simulink model "flexcan_s32k11x"  (Simulink 9.0)
settings: Solver=FixedStepDiscrete  StartTime=0.0  StopTime=10.0  FixedStep=0.1  RelTol=1e-3  EnableMultiTasking=on
InitFcn:
  | mbd_s32k_consistency_checks(bdroot(gcs));
undefined symbols (not defined in the file): LQFP, thumb
libraries: mbd_s32k1xx_ec_toolbox x9, simulink x1
Description:
  | This model tests the FlexCAN communication.
  | A numeric sequence with ID 0x3FF is send continuosly on FlexCAN0 to test the busload.
  | A received message with ID 0x3FE will toggle the PTD15 pin (Red LED) on each receive.
  | 
  | HW prerequisite:
  | - S32K116EVB-Q048/S32K118EVB
  | - Make sure that J107 has pin 1 and 2 connected and external power supply is provieded through J16.
  | 
  | Validation:
  | - The CAN Baudrate is set to 500 Kb/s.
  | - Any CAN analizer (USB to CAN device) can be used to observe CAN traffic via board CAN port J13.
settings Model: Creator=NXP MBDT Team  LastModifiedBy=nxf35401
settings DataIOCC: ExternalInput=off  InitialState=off  LimitDataPoints=on  SaveOutput=off  SignalLogging=off  SaveTime=off
settings OptimizationCC: DefaultParameterBehavior=Inlined  EnhancedBackFolding=on  PassReuseOutputArgsAs=Individual arguments  LifeSpan=auto  OptimizeBlockOrder=speed  DifferentSizesBufferReuse=on
settings DebuggingCC: SolverPrmCheckMsg=warning  InheritedTsInSrcMsg=none  SingleTaskRateTransMsg=error  ParameterTunabilityLossMsg=error  UnconnectedInputMsg=error  UnconnectedOutputMsg=error  UnconnectedLineMsg=error  AllowSymbolicDim=off  UnknownTsInhSupMsg=error  StateNameClashWarn=warning
settings HardwareCC: ProdLargestAtomicInteger=Long  ProdLargestAtomicFloat=Double  ProdIntDivRoundTo=Zero  ProdEndianess=LittleEndian  ProdHWDeviceType=ARM Compatible->ARM Cortex
settings SFSimCC: MATLABDynamicMemAlloc=off
settings RTWCC: SystemTargetFile=mbd_s32k.tlc  MakeCommand=mbd_s32k_make_rtw COPY_MDLREF_INCLUDES=0  TemplateMakefile=mbd_s32k.tmf  Description=Model Based Design Toolbox S32K14x Code Generation Target  GenerateReport=on  IncludeHyperlinkInReport=on  LaunchReport=on  GenerateTraceInfo=on  GenerateTraceReport=on  GenerateTraceReportSl=on  GenerateTraceReportSf=on  GenerateTraceReportEml=on
settings CodeAppCC: ForceParamTrailComments=on  IgnoreCustomStorageClasses=off  OperatorAnnotations=on  SimulinkDataObjDesc=on  SFDataObjDesc=on  InsertBlockDesc=on  StateflowObjectComments=off
settings STFCustomTargetCC: MultiwordLength=256  ModelReferenceCompliant=off  CombineOutputUpdateFcns=on  ERTCustomFileBanners=on  SupportContinuousTime=off  SupportNonInlinedSFcns=off  RemoveResetFunc=on  MATLABClassNameForMDSCustomization=Simulink.SoftwareTarget.ERTCustomization  GRTInterface=off  SystemTargetFile=mbd_s32k.tlc
settings ERTTargetCC: ModelReferenceCompliant=off  ParMdlRefBuildCompliant=off  CompOptLevelCompliant=off  ConcurrentExecutionCompliant=off  ModelStepFunctionPrototypeControlCompliant=off  CPPClassGenCompliant=off  UseToolchainInfoCompliant=off  InlinedParameterPlacement=NonHierarchical  ERTCustomFileTemplate=example_file_process.tlc

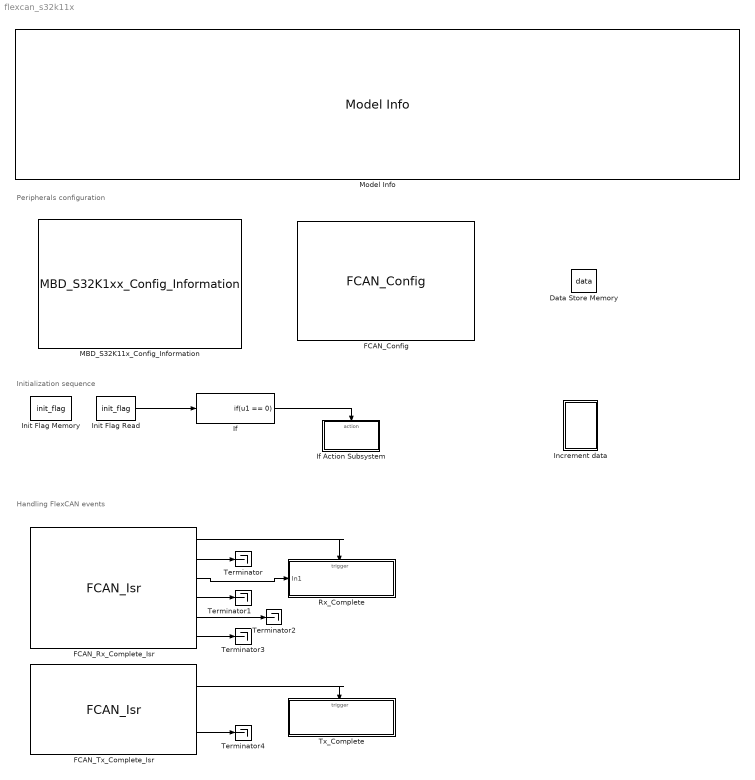
== system flexcan_s32k11x ==
  note: Peripherals configuration
  note: Handling FlexCAN events
  note: Initialization sequence
  Data Store Memory : DataStoreMemory  DataStoreName=data  ReadBeforeWriteMsg=warning  WriteAfterWriteMsg=warning  WriteAfterReadMsg=warning  ShowAdditionalParam=off  OutDataTypeStr=uint8
  FCAN_Config : mbd_s32k1xx_ec_toolbox/Communication Blocks/CAN Blocks/FCAN_Config  Priority=1  can_instance=0  can_mode=Normal mode  can_max_num_mb=16  can_rx=PTE4: [CAN0_RX | CAN Rx channel]  can_tx=PTE5: [CAN0_TX | CAN Tx Channel]  show_adv_opts=on  can_clk_src=Peripheral clock  bitrate=500  bitrate_adv_opts=off  can_presdiv=3  can_rjw=3  can_pseg1=6  can_pseg2=3  can_propseg=7  can_cbt_presdiv=1  can_cbt_rjw=3  can_cbt_pseg1=7  can_cbt_pseg2=7  can_cbt_propseg=6  can_fd_enable=off  can_payload=8  can_rxfifo_enable=off  can_fifo_id_filter_extended=off  can_fifo_id_filter_remote=off  can_num_id_filters=8  can_fifo_id_format=A  can_fifo_id_filter={'0x0', '0x0', '0x0', '0x0', '0x0', '0x0', '0x0', '0x0'}  can_pn_enable=off  can_wakeup_match=off  can_wakeup_timeout=off  can_timeout_en=off  can_match_timeout=1  can_multiple_matches_en=off  can_num_matches=1  can_idfilter_extendedid=off  can_idfilter_remoteframe=off  can_idfilter_type=Match exact  can_idfilter_id1=0  can_idfilter_id2=0  can_payloadfilter_enable=off  can_payloadfilter_dlclow=0  can_payloadfilter_dlchigh=0  can_payloadfilter_type=Match exact  can_payloadfilter_payload1_b0=0  can_payloadfilter_payload1_b1=0  can_payloadfilter_payload1_b2=0  can_payloadfilter_payload1_b3=0  can_payloadfilter_payload1_b4=0  can_payloadfilter_payload1_b5=0  can_payloadfilter_payload1_b6=0  can_payloadfilter_payload1_b7=0  can_payloadfilter_payload2_b0=0  can_payloadfilter_payload2_b1=0  can_payloadfilter_payload2_b2=0  can_payloadfilter_payload2_b3=0  can_payloadfilter_payload2_b4=0  can_payloadfilter_payload2_b5=0  can_payloadfilter_payload2_b6=0  can_payloadfilter_payload2_b7=0
  FCAN_Rx_Complete_Isr : mbd_s32k1xx_ec_toolbox/Communication Blocks/CAN Blocks/FCAN_Isr  can_instance=0  can_event=Rx Complete
  FCAN_Tx_Complete_Isr : mbd_s32k1xx_ec_toolbox/Communication Blocks/CAN Blocks/FCAN_Isr  can_instance=0  can_event=Tx Complete
  If : If  IfExpression=u1 == 0  ShowElse=off
  If Action Subsystem : Subsystem  TreatAsAtomicUnit=on
  Increment data : Subsystem
  Init Flag Memory : DataStoreMemory  DataStoreName=init_flag  ReadBeforeWriteMsg=warning  WriteAfterWriteMsg=warning  WriteAfterReadMsg=warning  ShowAdditionalParam=off  OutDataTypeStr=uint32
  Init Flag Read : DataStoreRead  DataStoreName=init_flag
  MBD_S32K11x_Config_Information : mbd_s32k1xx_ec_toolbox/MBD_S32K1xx_Config_Information  mbdt_ver=0  disp_str=|  config_params=[]  mcu_target_name=S32K116  mcu_target_package=48-LQFP  mcu_target_sram_size=17KB  mcu_system_clock_freq=40  mcu_xtal_freq=External 40  mcu_steptick_timer=LPIT Channel 0  mcu_steptick_prio=3  ds_import_enable=on  target_compiler=GCC  target_memory=FLASH  gcc_target_compile_opts=-mcpu=cortex-m0plus -mthumb -O1 -g -gstrict-dwarf  gcc_target_assemble_opts=-mcpu=cortex-m0plus -mthumb -g  gcc_target_link_opts=-mcpu=cortex-m0plus -mthumb  gcc_target_default_lcf=on  gcc_target_user_lcf=S32K116_17_flash.ld  ghs_target_compile_opts=-thumb -Ogeneral -Wundef -Wimplicit-int -Wshadow -Wtrigraphs --no_commons -c99 --gnu_asm -gdwarf-2 -G  ghs_target_assemble_opts=-thumb -preprocess_assembly_files -fsoft --gnu_asm  ghs_target_link_opts=-thumb  ghs_target_default_lcf=on  ghs_target_user_lcf=S32K116_17_flash.ld  iar_target_compile_opts=--thumb -Ol -e --debug --dlib_config normal  iar_target_assemble_opts=--thumb  iar_target_link_opts=--no_exceptions --vfe --inline  iar_target_default_lcf=on  iar_target_user_lcf=S32K116_17_flash.icf  pil_download_enable=off  rbl_download_enable=on  rbl_start_delay=5000  rbl_download_interface=OpenSDA  rbl_restart_request=off  rbl_com_port=Custom  rbl_com_port_custom=COM1  pil_download_rate=57600  pil_opensda_drive=Custom  pil_opensda_drive_custom=D  pil_uart_instance=0  pil_uart_rx=PTB0: [LPUART0_RX | Receive]  pil_uart_tx=PTB1: [LPUART0_TX | Transmit]  FTM_PWM_PcrCheckEnDis=on  FTM_Input_Edge_Inputs_PcrCheckEnDis=on  FTM_Dual_Edge_Inputs_PcrCheckEnDis=on  FTM_Quadrature_Inputs_PcrCheckEnDis=on  FTM_Hall_Sensor_Inputs_PcrCheckEnDis=on  LPTMR_PcrCheckEnDis=on  PIT_PcrCheckEnDis=on  RTC_PcrCheckEnDis=on  FlexCAN_PcrCheckEnDis=on  LIN_PcrCheckEnDis=on  FlexIO_PcrCheckEnDis=on  LPI2C_PcrCheckEnDis=on  LPSPI_PcrCheckEnDis=on  LPUART_PcrCheckEnDis=on  CMP_PcrCheckEnDis=on  GPIO_OutputPcrCheckEnDis=on  GPIO_InputPcrCheckEnDis=on  SBC_PcrCheckEnDis=on  AMMCLIB_PcrCheckEnDis=on  FM_PcrCheckEnDis=on  Profile_PcrCheckEnDis=on  ConfigParams_PcrCheckEnDis=on  ModelRef_PcrCheckEnDis=on  PDB0_PcrCheckEnDis=on  CSEc_PcrCheckEnDis=on  eDMA_PcrCheckEnDis=on  ADC_PcrCheckEnDis=on  WDOG_PcrCheckEnDis=on
      | Target : S32K144-64KB_SRAM
      | Package : 100-pin
      | System clock : 80 MHz
      | XTAL clock : External 8 MHz
      | Compiler : IAR
      | Target Type : FLASH
      | Download Code after build : off
      | Step Tick Interrupt Priority : 15
  Model Info : simulink/Model-Wide Utilities/Model Info  Frame=on  DisplayStringWithTags=|  HorizontalTextAlignment=Left  LeftAlignmentValue=0.02
      | Model Name: %<ModelName>
      | 
      | Description: %<Description>
  Rx_Complete : Subsystem  TreatAsAtomicUnit=on
      settings: RTWSystemCode=Nonreusable function
  Terminator{,1..4} (5 alike) : Terminator
  Tx_Complete : Subsystem  TreatAsAtomicUnit=on
      settings: RTWSystemCode=Nonreusable function
  wires:
  If/1 -> If Action Subsystem/Action
  Init Flag Read/1 -> If/1
  FCAN_Rx_Complete_Isr/1 -> Rx_Complete/Trigger
  FCAN_Rx_Complete_Isr/3 -> Rx_Complete/1(In1)
  FCAN_Tx_Complete_Isr/1 -> Tx_Complete/Trigger
  FCAN_Rx_Complete_Isr/2 -> Terminator/1
  FCAN_Rx_Complete_Isr/4 -> Terminator1/1
  FCAN_Rx_Complete_Isr/5 -> Terminator2/1
  FCAN_Tx_Complete_Isr/2 -> Terminator4/1
  FCAN_Rx_Complete_Isr/6 -> Terminator3/1

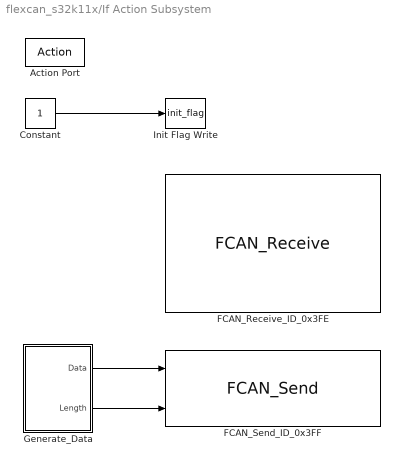
== system flexcan_s32k11x/If Action Subsystem ==
  Action Port : ActionPort  ActionType=then
  Constant : Constant  OutDataTypeStr=uint32
  FCAN_Receive_ID_0x3FE : mbd_s32k1xx_ec_toolbox/Communication Blocks/CAN Blocks/FCAN_Receive  can_instance=0  can_mode=Non-blocking  can_timeout_ms=0  can_mb_idx=14  can_extended_id=off  can_is_remote=off  can_id=3FE  can_msg_mask=FFFFFFFF  show_adv_opts=off  can_use_rxfifo=off  can_fd_enable=off
  FCAN_Send_ID_0x3FF : mbd_s32k1xx_ec_toolbox/Communication Blocks/CAN Blocks/FCAN_Send  Priority=2  can_instance=0  can_mode=Non-blocking  can_timeout_ms=0  can_mb_idx=15  can_extended_id=off  can_is_remote=off  can_id=3FF  show_adv_opts=off  can_fd_enable=off  can_enable_brs=off  can_fd_padding=0
  Generate_Data : Subsystem
  Init Flag Write : DataStoreWrite  DataStoreName=init_flag
  wires:
  Generate_Data/1(Data) -> FCAN_Send_ID_0x3FF/1
  Constant/1 -> Init Flag Write/1
  Generate_Data/2(Length) -> FCAN_Send_ID_0x3FF/2

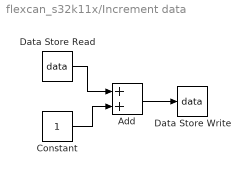
== system flexcan_s32k11x/Increment data ==
  Add : Sum
  Constant : Constant  OutDataTypeStr=uint8
  Data Store Read : DataStoreRead  DataStoreName=data
  Data Store Write : DataStoreWrite  DataStoreName=data
  wires:
  Add/1 -> Data Store Write/1
  Data Store Read/1 -> Add/1
  Constant/1 -> Add/2

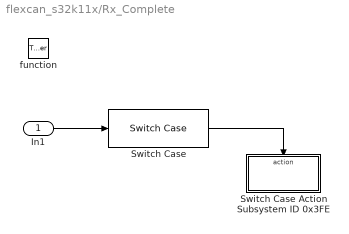
== system flexcan_s32k11x/Rx_Complete ==
  In1 : Inport
  function : TriggerPort  TriggerType=function-call  VariantControl=Variant
  Switch Case : SwitchCase  CaseConditions={hex2dec('3FE')}  ShowDefaultCase=off
  Switch Case Action Subsystem ID 0x3FE : Subsystem  TreatAsAtomicUnit=on
  wires:
  In1/1 -> Switch Case/1
  Switch Case/1 -> Switch Case Action Subsystem ID 0x3FE/Action

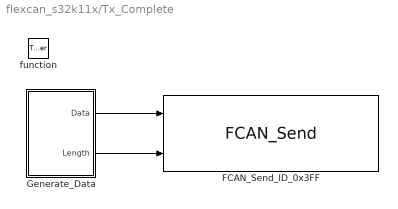
== system flexcan_s32k11x/Tx_Complete ==
  function : TriggerPort  TriggerType=function-call  VariantControl=Variant
  FCAN_Send_ID_0x3FF : mbd_s32k1xx_ec_toolbox/Communication Blocks/CAN Blocks/FCAN_Send  Priority=2  can_instance=0  can_mode=Non-blocking  can_timeout_ms=0  can_mb_idx=15  can_extended_id=off  can_is_remote=off  can_id=3FF  show_adv_opts=off  can_fd_enable=off  can_enable_brs=off  can_fd_padding=0
  Generate_Data : Subsystem
  wires:
  Generate_Data/1(Data) -> FCAN_Send_ID_0x3FF/1
  Generate_Data/2(Length) -> FCAN_Send_ID_0x3FF/2

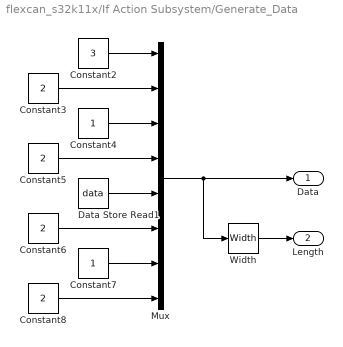
== system flexcan_s32k11x/If Action Subsystem/Generate_Data ==
  Constant2 : Constant  Value=3  OutDataTypeStr=uint8
  Constant{3,5..6,8} (4 alike) : Constant  Value=2  OutDataTypeStr=uint8
  Constant4 : Constant  OutDataTypeStr=uint8
  Constant7 : Constant  OutDataTypeStr=uint8
  Data Store Read1 : DataStoreRead  DataStoreName=data
  Mux : Mux  Inputs=8
  Width : Width  DataType=uint8
  Data : Outport
  Length : Outport  Port=2
  wires:
  Mux/1 -> Width/1, Data/1
  Constant2/1 -> Mux/1
  Constant3/1 -> Mux/2
  Constant5/1 -> Mux/4
  Data Store Read1/1 -> Mux/5
  Constant4/1 -> Mux/3
  Constant6/1 -> Mux/6
  Constant7/1 -> Mux/7
  Constant8/1 -> Mux/8
  Width/1 -> Length/1

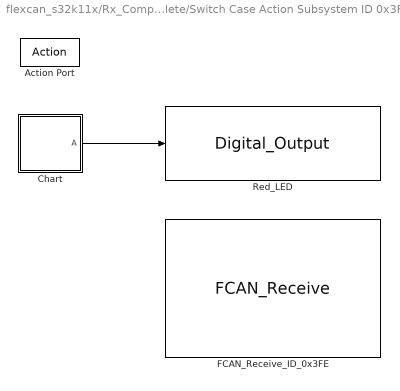
== system flexcan_s32k11x/Rx_Complete/Switch Case Action Subsystem ID 0x3FE ==
  Action Port : ActionPort  ActionType=case
  Chart : Stateflow chart  TreatAsAtomicUnit=on
  FCAN_Receive_ID_0x3FE : mbd_s32k1xx_ec_toolbox/Communication Blocks/CAN Blocks/FCAN_Receive  can_instance=0  can_mode=Non-blocking  can_timeout_ms=0  can_mb_idx=14  can_extended_id=off  can_is_remote=off  can_id=3FE  can_msg_mask=FFFFFFFF  show_adv_opts=off  can_use_rxfifo=off  can_fd_enable=off
  Red_LED : mbd_s32k1xx_ec_toolbox/GPIO Blocks/Digital_Output  gpio_pin=PTD15: [PTD15 | Port D I/O]  init_val=Low  drive_strength=Low
  wires:
  Chart/1(" A") -> Red_LED/1

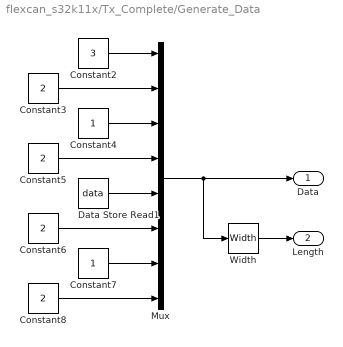
== system flexcan_s32k11x/Tx_Complete/Generate_Data ==
  Constant2 : Constant  Value=3  OutDataTypeStr=uint8
  Constant{3,5..6,8} (4 alike) : Constant  Value=2  OutDataTypeStr=uint8
  Constant4 : Constant  OutDataTypeStr=uint8
  Constant7 : Constant  OutDataTypeStr=uint8
  Data Store Read1 : DataStoreRead  DataStoreName=data
  Mux : Mux  Inputs=8
  Width : Width  DataType=uint8
  Data : Outport
  Length : Outport  Port=2
  wires:
  Mux/1 -> Width/1, Data/1
  Constant2/1 -> Mux/1
  Constant3/1 -> Mux/2
  Constant5/1 -> Mux/4
  Data Store Read1/1 -> Mux/5
  Constant4/1 -> Mux/3
  Constant6/1 -> Mux/6
  Constant7/1 -> Mux/7
  Constant8/1 -> Mux/8
  Width/1 -> Length/1

== stateflow chart Rx_Complete/Switch Case Action Subsystem ID 0x3FE/Chart ==
  state A
  state A1
  (default) -> A
  A -> A1
  A1 -> A
  data: A output boolean [0..1]
